simulink model "x35BusNetworkElectricityTransmissionModel"  (R2023b)
settings: Solver=VariableStepAuto  StartTime=0.0  StopTime=0.8  RelTol=1e-3
model workspace (MAT data in the model file):
  Compensation_Ki = 30
  Compensation_Kp = 3
  DC_Ki = 400
  DC_Kp = 8
  F = 0.01
  Flux_min = 0.5
  Grid_Freq_PWM = 2700
  Grid_Ireg_Ki = 5
  Grid_Ireg_Kp = 0.83
  Grid_Ireg_lim = 1.1
  Grid_Modindex_Upper = 1.1
  Grid_conv_Imax = 0.8
  H = 0.685
  Idref_max = 0.9
  Iqref_Tc = 0.3
  Ki_Var = 0.05
  Ki_Vreg = 20
  Ksh = 1.1
  L_pu = 0.3
  Llr = 0.16
  Lls = 0.18
  Lm = 2.9
  Nb_wt = 6
  P_mech = 1080000
  Pitch_Ki = 0
  Pitch_Kp = 150
  Pitch_Max = 27
  Pitch_Tc = 0.01
  Pitch_rate = 10
  Q_Filt = 50
  R_pu = 0.003
  Rotor_Freq_PWM = 1620
  Rotor_Ireg_Ki = 8
  Rotor_Ireg_Kp = 0.6
  Rotor_Ireg_lim = 0.1
  Rotor_Modindex_Upper = 2
  Rr = 0.016
  Rs = 0.023
  T_set = 0.0001
  Tp = 5e-05
  Ts = 5e-06
  Var_C_Filt = 720000
  Var_reg_max = 1.1
  Var_reg_min = 0.9
  WT_Coeff = [0.645 116 0.4 5 21 0.00912 0.08 0.035]
  WT_H = 4.32
  WT_IGBTRon = 5.931
  WT_Param = [91.204 10143]
  Wind_Freq_Filt = 10000
  Wind_Freq_nom = 60
  Wind_P_nom = 1200000
  Wind_Rotor_V_nom = 1950
  Wind_V_nom = 500
  Zeta_Filt = 0.707106781187
  init = [-0.2 0 0 0 0 0 0 0]
  p = 3
  torque0 = 0.83
  v_Ki = 0.1
  v_Kp = 3.6
  v_Max = 1.2
  v_Min = 0.7
  v_T = 5
  vreg_max = 1
  wind_VDC_nom = 1150
  wt0 = 1.2
undefined symbols (not defined in the file): D1, D11, Delta, DiscIntNeverNeededParam, Ion, Lithium, P, Q
libraries: powerlib_extras x144, spsSeriesRLCBranchLib x67, spsLoadFlowBusLib x43, spsThreePhaseTransformerTwoWindingsLib x32, spsThreePhaseSeriesRLCLoadLib x31, spsThreePhaseVIMeasurementLib x26, simulink_extras x26, spsDistributedParametersLineLib x22, spsGenericPowerSystemStabilizerLib x20, spsSynchronousMachinepuStandardLib x10, spsExcitationSystemLib x10, spsHydraulicTurbineandGovernorLib x10
(part 1 of 16)
settings Model: Creator=3.22  LastModifiedBy=3.22

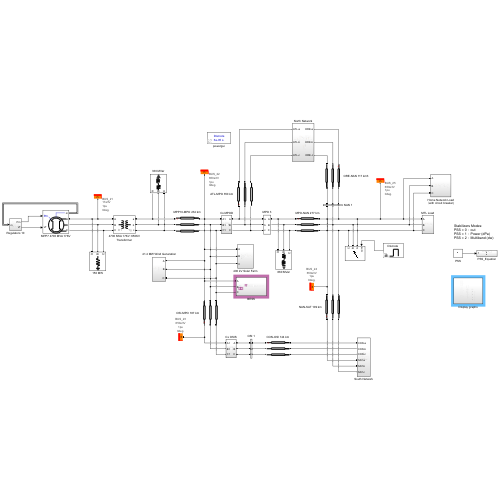
[thumbnail: Simulink's stored preview of the top-level diagram]
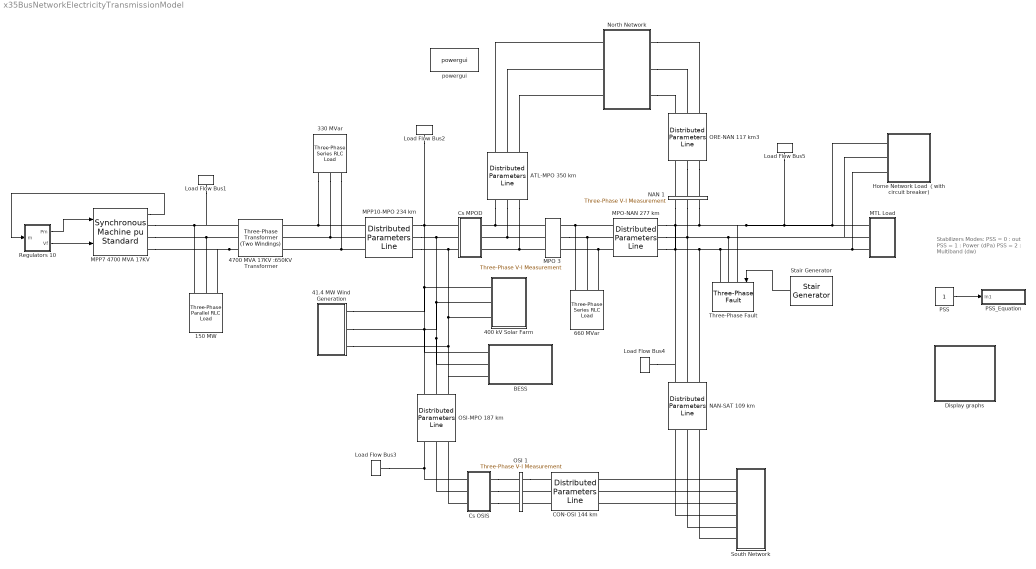
== system x35BusNetworkElectricityTransmissionModel ==
  note: Stabilizers Modes:
      | PSS = 0 :  out
      | PSS = 1 :  Power (dPa)
      | PSS = 2 :  Multiband (dw)
  " 41.4 MW Wind Generation" : Subsystem
  150 MW : spsThreePhaseParallelRLCLoadLib/Three-Phase Parallel RLC Load  LConnTagsString=A|B|C  Configuration=Y (grounded)  NominalVoltage=17000  Vabc=[1e3 1e3 1e3]  Vabcp=[1e3 1e3 1e3]  NominalFrequency=60  UnbalancedPower=off  ActivePower=150e6  InductivePower=0  CapacitivePower=0  Pabc=[10e3 9e3 11e3]  QLabc=[100 90 110]  QCabc=[100 90 110]  Pabcp=[10e3 9e3 11e3]  QLabcp=[100 90 110]  QCabcp=[100 90 110]  Measurements=None  LoadType=constant Z
  330 MVar : spsThreePhaseSeriesRLCLoadLib/Three-Phase Series RLC Load  LConnTagsString=A|B|C  Configuration=Y (grounded)  NominalVoltage=650e3  Vabc=[1e3 1e3 1e3]  Vabcp=[1e3 1e3 1e3]  NominalFrequency=60  UnbalancedPower=off  ActivePower=1100e3  InductivePower=330e6  CapacitivePower=0  Pabc=[10e3 9e3 11e3]  QLabc=[100 90 110]  QCabc=[100 90 110]  Pabcp=[10e3 9e3 11e3]  QLabcp=[100 90 110]  QCabcp=[100 90 110]  Measurements=None  LoadType=constant Z
  400 kV Solar Farm : Subsystem
  "4700 MVA 17KV :650KV Transformer " : spsThreePhaseTransformerTwoWindingsLib/Three-Phase Transformer (Two Windings)  Winding1Connection=Delta (D1)  Winding2Connection=Yg  CoreType=Three single-phase transformers  SetSaturation=off  Hysteresis=off  DataFile='hysteresis'  SetInitialFlux=off  Measurements=None  UNITS=pu  NominalPower=[ 4700e6 , 60 ]  Winding1=[ 17e3 , 0.002 , 0.08 ]  Winding2=[ 650e3 , 0.002 , 0.08 ]  Rm=500  Lm=500  L0=0.5  Saturation=[ 0,0 ; 0.0024,1.2 ; 1.0,1.52 ]  InitialFluxes=[ 0.8 , -0.8 , 0.7 ]  BreakLoop=off  DiscreteSolver=Trapezoidal iterative  DataType=off  TransfoNumber=1
  660 MVar : spsThreePhaseSeriesRLCLoadLib/Three-Phase Series RLC Load  LConnTagsString=A|B|C  Configuration=Y (grounded)  NominalVoltage=650e3  Vabc=[1e3 1e3 1e3]  Vabcp=[1e3 1e3 1e3]  NominalFrequency=60  UnbalancedPower=off  ActivePower=2200e3  InductivePower=660e6  CapacitivePower=0  Pabc=[10e3 9e3 11e3]  QLabc=[100 90 110]  QCabc=[100 90 110]  Pabcp=[10e3 9e3 11e3]  QLabcp=[100 90 110]  QCabcp=[100 90 110]  Measurements=None  LoadType=constant Z
  ATL-MPO 350 km : spsDistributedParametersLineLib/Distributed Parameters Line  Phases=3  Length=350  Frequency=60  Resistance=[0.01273 0.3864]/6  Inductance="[0.9337e-3  4.1264e-3]/6"  Capacitance=[12.74e-9 7.751e-9]*6  x1=[-0.00198 -8.81886184233511e-10 -287572.775174279 -158100.693471797;-0.00192 -9.46737266554495e-10 -283923.339530845 -164564.466267701;-0.00186 -1.01110398059622e-09 -280128.643460608 -170944.044841861;-0.0018 -1.07495339515841e-09 -276190.628400193 -177236.165283997;-0.00174 -1.13825284370079e-09 -272111.309110873 -183437.608429026;-0.00168 -1.20096994105583e-09 -267892.772647773 -189545.201504045;-0.00162 -1.26307259999766e-09 -263537.177292097 -195555.819751582;-0.00156 -1.32452904765843e-09 -259046.751446911 -201466.388028279;-0.0015 -1.38530784178394e-09 -254423.792497051 -207273.882378189;-0.00144 -1.44537788682004e-09 -249670.665633739 -212975.331579893;-0.00138 -1.50470844982173e-09 -244789.802644505 -218567.81866663;-0.00132 -1.56326917617668e-09 -239783.700669043 -224048.482418667;-0.00126 -1.62103010513521e-09 -234654.920921625 -229414.51882716;-0.0012 -1.67796168513875e-09 -229406.087380739 -234663.182528727;-0.00114 -1.73403478893901e-09 -224039.885446612 -239791.788210036;-0.00108 -1.78922072849997e-09 -218559.060567309 -244797.711981654;-0.00102 -1.84349126967524e-09 -212966.416834113 -249678.39272048;-0.00096 -1.89681864665313e-09 -207264.815546898 -254431.333380064;-0.0009 -1.94917557616222e-09 -201457.173750235 -259054.102268141;-0.00084 -2.00053527142992e-09 -195546.462740982 -263544.334290727;-0.00078 -2.05087145588711e-09 -189535.706548106 -267899.732162151;-0.00072 -2.10015837661173e-09 -183427.980385544 -272118.067580383;-0.00066 -2.1483708175044e-09 -177226.409078857 -276197.182367078;-0.0006 -2.19548411218952e-09 -170934.165466518 -280134.989571736;-0.00054 -2.24147415663495e-09 -164554.468776626 -283929.474539429;-0.00048 -2.28631742148417e-09 -158090.582979891 -287578.695941535;-0.00042 -2.32999096409427e-09 -151545.815119725 -291080.786768954;-0.00036 -2.37247244027385e-09 -144923.513620299 -294433.955287307;-0.0003 -2.41374011571475e-09 -138227.066573427 -297636.485953622;-0.00024 -2.45377287711165e-09 -131459.900005152 -300686.740294032;-0.00018 -2.49255024296411e-09 -124625.476122936 -303583.157742056;-0.00012 -2.53005237405524e-09 -117727.291544321 -306324.256437008;-6e-05 -2.56626008360181e-09 -110768.875508002 -308908.633982145]  x2=[-0.00198 1.54433518898386e-08 -267682.446603461 -181667.296939203;-0.00192 1.64654785965534e-08 -263505.082563477 -187675.172287145;-0.00186 1.74791812601711e-08 -259192.904454239 -193587.029549106;-0.0018 1.84839412516781e-08 -254748.118465748 -199399.844109673;-0.00174 1.94792445172967e-08 -250172.998632646 -205110.642025508;-0.00168 2.04645818414852e-08 -245469.885670778 -210716.501546873;-0.00162 2.14394491074616e-08 -240641.185779639 -216214.554612454;-0.00156 2.24033475551191e-08 -235689.369411317 -221601.98831671;-0.0015 2.33557840362012e-08 -230616.970006566 -226876.046349009;-0.00144 2.42962712666051e-08 -225426.582698647 -232034.030403808;-0.00138 2.52243280756855e-08 -220120.862985616 -237073.301561157;-0.00132 2.61394796524304e-08 -214702.525371715 -241991.281636816;-0.00126 2.70412577883831e-08 -209174.341978588 -246785.454501306;-0.0012 2.79292011171863e-08 -203539.141127007 -251453.367367201;-0.00114 2.88028553506256e-08 -197799.805889854 -255992.632044027;-0.00108 2.96617735110519e-08 -191959.272617088 -260400.9261601;-0.00102 3.05055161600635e-08 -186020.529433451 -264675.994350693;-0.00096 3.13336516233304e-08 -179986.614709693 -268815.649411926;-0.0009 3.21457562114475e-08 -173860.615508078 -272817.773419778;-0.00084 3.29414144367015e-08 -167645.666002995 -276680.318813656;-0.00078 3.37202192256424e-08 -161344.945877449 -280401.309443964;-0.00072 3.44817721273494e-08 -154961.67869628 -283978.84158314;-0.00066 3.52256835172862e-08 -148499.130256927 -287411.084899637;-0.0006 3.59515727966398e-08 -141960.606918587 -290696.283394352;-0.00054 3.66590685870419e-08 -135349.453910617 -293832.756299034;-0.00048 3.73478089205732e-08 -128669.053621055 -296818.898936187;-0.00042 3.80174414249525e-08 -121922.823866131 -299653.183540063;-0.00036 3.86676235038173e-08 -115114.216141641 -302334.160038285;-0.0003 3.9298022512002e-08 -108246.713857108 -304860.456793738;-0.00024 3.99083159257256e-08 -101323.830553596 -307230.781306322;-0.00018 4.04981915076007e-08 -94349.1081061232 -309443.920874218;-0.00012 4.106734746638e-08 -87326.1149115726 -311498.743214328;-6e-05 4.16154926113581e-08 -80258.4440630321 -313394.197041575]  x3=[-0.00198 -4.6655895685918e-10 -8241.46905294037 -3030.79596300684;-0.00192 -4.60608629980999e-10 -8170.81094503147 -3216.42300046448;-0.00186 -4.54422647216651e-10 -8095.97249926386 -3400.40445648242;-0.0018 -4.48004173429221e-10 -8016.99200436926 -3582.64620274818;-0.00174 -4.413564924285e-10 -7933.90986822824 -3763.05500101691;-0.00168 -4.34483005290922e-10 -7846.76859719684 -3941.53855081387;-0.00162 -4.27387228619515e-10 -7755.6127743595 -4118.00553665697;-0.00156 -4.20072792744737e-10 -7660.48903671955 -4292.36567477553;-0.0015 -4.12543439867139e-10 -7561.44605133885 -4464.52975930106;-0.00144 -4.04803022142778e-10 -7458.53449043883 -4634.40970790672;-0.00138 -3.9685549971239e-10 -7351.80700547563 -4801.91860687177;-0.00132 -3.88704938675302e-10 -7241.31820020265 -4966.97075554829;-0.00126 -3.80355509009146e-10 -7127.12460273427 -5129.4817102072;-0.0012 -3.71811482436419e-10 -7009.28463662502 -5289.36832724124;-0.00114 -3.63077230238992e-10 -6887.85859097897 -5446.54880570278;-0.00108 -3.54157221021679e-10 -6762.90858960479 -5600.94272915467;-0.00102 -3.45056018426017e-10 -6634.49855923199 -5752.4711068128;-0.00096 -3.35778278795427e-10 -6502.69419680484 -5901.05641395925;-0.0009 -3.26328748792936e-10 -6367.56293587064 -6046.62263160532;-0.00084 -3.16712262972701e-10 -6229.17391207941 -6189.09528538433;-0.00078 -3.06933741306559e-10 -6087.59792781285 -6328.401483654;-0.00072 -2.96998186666881e-10 -5942.90741596056 -6464.46995478922;-0.00066 -2.86910682267009e-10 -5795.17640286195 -6597.2310836459;-0.0006 -2.76676389060589e-10 -5644.4804704331 -6726.61694717737;-0.00054 -2.66300543101134e-10 -5490.89671749756 -6852.56134918508;-0.00048 -2.5578845286316e-10 -5334.50372034124 -6974.99985418576;-0.00042 -2.45145496526274e-10 -5175.3814925113 -7093.86982037787;-0.00036 -2.34377119223597e-10 -5013.61144387974 -7209.11043169023;-0.0003 -2.23488830255934e-10 -4849.27633899261 -7320.66272889669;-0.00024 -2.12486200273114e-10 -4682.46025472612 -7428.46963978076;-0.00018 -2.0137485842394e-10 -4513.24853727139 -7532.47600833477;-0.00012 -1.90160489476217e-10 -4341.72775846975 -7632.62862297877;-6e-05 -1.78848830908316e-10 -4167.98567152098 -7728.87624378449]  x4=[-0.00198 4.4437183156576e-10 -5640.56823399598 -1579.41875960243;-0.00192 4.46231326418624e-10 -5603.40220789252 -1706.59093166833;-0.00186 4.47862521079487e-10 -5563.36937768053 -1832.88998027941;-0.0018 4.49264580999017e-10 -5520.49022489568 -1958.25128850867;-0.00174 4.50436788857453e-10 -5474.78668730484 -2082.6107191944;-0.00168 4.51378544931595e-10 -5426.28214768235 -2205.90464775398;-0.00162 4.52089367401633e-10 -5375.00142184694 -2328.06999473533;-0.00156 4.52568892597658e-10 -5320.9707459655 -2449.04425808958;-0.0015 4.52816875185718e-10 -5264.2177631302 -2568.76554514826;-0.00144 4.52833188293339e-10 -5204.77150921571 -2687.17260428872;-0.00138 4.52617823574434e-10 -5142.662398024 -2804.20485627158;-0.00132 4.52170891213572e-10 -5077.92220572397 -2919.80242523422;-0.00126 4.51492619869608e-10 -5010.58405459429 -3033.90616932437;-0.0012 4.50583356558695e-10 -4940.68239607732 -3146.45771095815;-0.00114 4.49443566476743e-10 -4868.25299315321 -3257.39946668715;-0.00108 4.48073832761419e-10 -4793.33290204283 -3366.67467665917;-0.00102 4.46474856193802e-10 -4715.96045324916 -3474.22743365762;-0.00096 4.44647454839849e-10 -4636.17523194667 -3580.00271170466;-0.0009 4.4259256363186e-10 -4554.01805772885 -3683.94639421356;-0.00084 4.40311233890147e-10 -4469.53096372412 -3786.00530167567;-0.00078 4.37804632785159e-10 -4382.75717509091 -3886.12721886811;-0.00072 4.35074042740339e-10 -4293.74108690288 -3984.260921568;-0.00066 4.3212086077601e-10 -4202.52824143558 -4080.35620275974;-0.0006 4.28946597794631e-10 -4109.16530486617 -4174.36389832184;-0.00054 4.25552877807799e-10 -4013.70004339815 -4266.23591218018;-0.00048 4.21941437105368e-10 -3916.18129882327 -4355.92524091487;-0.00042 4.18114123367132e-10 -3816.6589635332 -4443.38599780806;-0.00036 4.14072894717521e-10 -3715.18395499364 -4528.57343632044;-0.0003 4.09819818723784e-10 -3611.808189694 -4611.44397298439;-0.00024 4.0535707133819e-10 -3506.58455658597 -4691.95520970207;-0.00018 4.00686935784761e-10 -3399.56689002456 -4770.0659554371;-0.00012 3.95811801391141e-10 -3290.80994222544 -4845.73624728864;-6e-05 3.90734162366169e-10 -3180.3693552527 -4918.92737093716]  x5=0.0019793954844851  V1=[4.219e-16 0.0001256 0.0001256;377 377 377;2.896 1.02 -0.5506]  V2=[3.447e-16 8.016e-05 8.016e-05;377 377 377;2.788 1.015 -0.5555]  I1=[4.128e-19 5.188e-07 5.188e-07;377 377 377;2.697 1.572 0.0007381]  I2=[5.884e-19 5.436e-07 5.436e-07;377 377 377;2.289 0.05248 -1.518]  nHarmo=1  Measurements=None  Decoupling=off  VsMag0=0  VrMag0=0  VsAngle0=0  VrAngle0=0  IsMag0=0  IrMag0=0  IsAngle0=0  IrAngle0=0
      settings: LibrarySourceBlock=sps_lib/Power Grid Elements/Distributed Parameters Line
  BESS : Subsystem
  CON-OSI 144 km : spsDistributedParametersLineLib/Distributed Parameters Line  Phases=3  Length=144  Frequency=60  Resistance=[0.01273 0.3864]/6  Inductance="[0.9337e-3  4.1264e-3]/6"  Capacitance=[12.74e-9 7.751e-9]*6  x1=[-0.00084 1.00465090106322e-08 0 0;-0.00078 1.0437043643029e-08 0 0;-0.00072 1.08222384910436e-08 0 0;-0.00066 1.12018964818742e-08 0 0;-0.0006 1.15758233754775e-08 0 0;-0.00054 1.19438278639452e-08 -161808.366832188 -299092.068846077;-0.00048 1.23057216693812e-08 -155002.244278101 -302675.302733702;-0.00042 1.26613196402275e-08 -148116.819711728 -306103.682343652;-0.00036 1.30104398459916e-08 -141155.615843508 -309375.45365357;-0.0003 1.33529036703253e-08 -134122.194153965 -312488.942764797;-0.00024 1.36885359024078e-08 -127020.1530716 -315442.556758774;-0.00018 1.40171648265877e-08 -119853.126131861 -318234.784512005;-0.00012 1.43386223102348e-08 -112624.780118162 -320864.197469177;-6e-05 1.46527438897608e-08 -105338.813185888 -323329.450374036]  x2=[-0.00084 1.696883336304e-08 0 0;-0.00078 1.76603541306248e-08 0 0;-0.00072 1.83428395347105e-08 0 0;-0.00066 1.90159404031536e-08 0 0;-0.0006 1.96793123651122e-08 0 0;-0.00054 2.0332616027233e-08 -156405.712657969 -298820.407534756;-0.00048 2.09755171472907e-08 -149607.117035199 -302281.515873199;-0.00042 2.16076868051928e-08 -142731.979646933 -305587.971402601;-0.00036 2.22288015712613e-08 -135783.817940495 -308738.082479218;-0.0003 2.28385436717049e-08 -128766.186723802 -311730.237448014;-0.00024 2.34366011511983e-08 -121682.676346656 -314562.905467219;-0.00018 2.40226680324841e-08 -114536.910863854 -317234.637291533;-0.00012 2.45964444729166e-08 -107332.546181055 -319744.066013586;-6e-05 2.51576369178668e-08 -100073.268184352 -322089.907763276]  x3=[-0.00084 -2.32474030583707e-10 0 0;-0.00078 -2.23427423220123e-10 0 0;-0.00072 -2.14266506258355e-10 0 0;-0.00066 -2.04995966592796e-10 0 0;-0.0006 -1.95620547202837e-10 0 0;-0.00054 -1.86145044726278e-10 -4133.07539991967 -6898.70820759528;-0.00048 -1.76574307005272e-10 -3975.98619314656 -6990.42432957894;-0.00042 -1.66913230606083e-10 -3816.86279836927 -7078.5640213074;-0.00036 -1.57166758313915e-10 -3655.78662605681 -7163.08218888573;-0.0003 -1.47339876604086e-10 -3492.84008575529 -7243.93559125769;-0.00024 -1.37437613090858e-10 -3328.10654392563 -7321.08286232862;-0.00018 -1.27465033955217e-10 -3161.67028129177 -7394.48453212913;-0.00012 -1.17427241352923e-10 -2993.61644972104 -7464.10304700863;-6e-05 -1.07329370804146e-10 -2824.03102865897 -7529.90278884852]  x4=[-0.00084 3.81260191027999e-10 0 0;-0.00078 3.81331768701559e-10 0 0;-0.00072 3.8120824999605e-10 0 0;-0.00066 3.80889698105924e-10 0 0;-0.0006 3.80376276008215e-10 0 0;-0.00054 3.79668246379155e-10 -4123.74727696322 -5625.68716163841;-0.00048 3.78765971459785e-10 -3995.45299481996 -5717.51781638891;-0.00042 3.77669912870626e-10 -3865.11456509707 -5806.42328337696;-0.00036 3.76380631375504e-10 -3732.79867134357 -5892.35807692286;-0.0003 3.74898786594656e-10 -3598.57300881562 -5975.27823119836;-0.00024 3.73225136667253e-10 -3462.50624984237 -6055.14132272033;-0.00018 3.71360537863524e-10 -3324.66800869195 -6131.90649205544;-0.00012 3.6930594414667e-10 -3185.12880595548 -6205.53446472462;-6e-05 3.67062406684801e-10 -3043.96003246747 -6275.98757129655]  x5=0.000814379856473869  V1=[3.066e-13 0.3294 0.3294;377 377 377;-0.5534 -1.851 2.861]  V2=[2.167e-13 0.2213 0.2213;377 377 377;-0.5727 -1.852 2.86]  I1=[4.19e-16 0.002316 0.002316;377 377 377;0.2564 -0.79 -2.361]  I2=[5.677e-16 0.002387 0.002387;377 377 377;-1.374 -3.038 1.674]  nHarmo=1  Measurements=None  Decoupling=off  VsMag0=0  VrMag0=0  VsAngle0=0  VrAngle0=0  IsMag0=0  IrMag0=0  IsAngle0=0  IrAngle0=0
      settings: LibrarySourceBlock=sps_lib/Power Grid Elements/Distributed Parameters Line
  Cs MPOD : Subsystem
  Cs OSIS : Subsystem
  Display graphs : Subsystem
  Home Network Load （with circuit breaker) : Subsystem
  Load Flow Bus1 : spsLoadFlowBusLib/Load Flow Bus  LConnTagsString=a  Phases=single  Connectors=on one side  ID=BUS_21  Vbase=17e3  Vref=1  Vangle=0  VLF=1  VLFb=1  VLFc=1  angleLF=0  angleLFb=0  angleLFc=0
  Load Flow Bus2 : spsLoadFlowBusLib/Load Flow Bus  LConnTagsString=a  Phases=single  Connectors=on one side  ID=BUS_22  Vbase=650e3  Vref=1  Vangle=0  VLF=1  VLFb=1  VLFc=1  angleLF=0  angleLFb=0  angleLFc=0
  Load Flow Bus3 : spsLoadFlowBusLib/Load Flow Bus  LConnTagsString=a  Phases=single  Connectors=on one side  ID=BUS_23  Vbase=650e3  Vref=1  Vangle=0  VLF=1  VLFb=1  VLFc=1  angleLF=0  angleLFb=0  angleLFc=0
  Load Flow Bus4 : spsLoadFlowBusLib/Load Flow Bus  LConnTagsString=a  Phases=single  Connectors=on one side  ID=BUS_24  Vbase=650e3  Vref=1  Vangle=0  VLF=1  VLFb=1  VLFc=1  angleLF=0  angleLFb=0  angleLFc=0
  Load Flow Bus5 : spsLoadFlowBusLib/Load Flow Bus  LConnTagsString=a  Phases=single  Connectors=on one side  ID=BUS_25  Vbase=650e3  Vref=1  Vangle=0  VLF=1  VLFb=1  VLFc=1  angleLF=0  angleLFb=0  angleLFc=0
  MPO 3 : spsThreePhaseVIMeasurementLib/Three-Phase V-I Measurement  VoltageMeasurement=no  SetLabelV=off  LabelV=Vabc_MPO3  Vpu=off  VpuLL=off  CurrentMeasurement=no  SetLabelI=off  LabelI=Iabc  Ipu=off  Pbase=100e6  Vbase=500e3  OutputType=Complex  PhasorSimulation=off  PSBequivalent=0
  MPO-NAN 277 km : spsDistributedParametersLineLib/Distributed Parameters Line  Phases=3  Length=277  Frequency=60  Resistance=[0.01273 0.3864]/6  Inductance="[0.9337e-3  4.1264e-3]/6"  Capacitance=[12.74e-9 7.751e-9]*6  x1=[-0.00162 -1.26307259999766e-09 -263537.177292097 -195555.819751582;-0.00156 -1.32452904765843e-09 -259046.751446911 -201466.388028279;-0.0015 -1.38530784178394e-09 -254423.792497051 -207273.882378189;-0.00144 -1.44537788682004e-09 -249670.665633739 -212975.331579893;-0.00138 -1.50470844982173e-09 -244789.802644505 -218567.81866663;-0.00132 -1.56326917617668e-09 -239783.700669043 -224048.482418667;-0.00126 -1.62103010513521e-09 -234654.920921625 -229414.51882716;-0.0012 -1.67796168513875e-09 -229406.087380739 -234663.182528727;-0.00114 -1.73403478893901e-09 -224039.885446612 -239791.788210036;-0.00108 -1.78922072849997e-09 -218559.060567309 -244797.711981654;-0.00102 -1.84349126967524e-09 -212966.416834113 -249678.39272048;-0.00096 -1.89681864665313e-09 -207264.815546898 -254431.333380064;-0.0009 -1.94917557616222e-09 -201457.173750235 -259054.102268141;-0.00084 -2.00053527142992e-09 -195546.462740982 -263544.334290727;-0.00078 -2.05087145588711e-09 -189535.706548106 -267899.732162151;-0.00072 -2.10015837661173e-09 -183427.980385544 -272118.067580383;-0.00066 -2.1483708175044e-09 -177226.409078857 -276197.182367078;-0.0006 -2.19548411218952e-09 -170934.165466518 -280134.989571736;-0.00054 -2.24147415663495e-09 -164554.468776626 -283929.474539429;-0.00048 -2.28631742148417e-09 -158090.582979891 -287578.695941535;-0.00042 -2.32999096409427e-09 -151545.815119725 -291080.786768954;-0.00036 -2.37247244027385e-09 -144923.513620299 -294433.955287307;-0.0003 -2.41374011571475e-09 -138227.066573427 -297636.485953622;-0.00024 -2.45377287711165e-09 -131459.900005152 -300686.740294032;-0.00018 -2.49255024296411e-09 -124625.476122936 -303583.157742056;-0.00012 -2.53005237405524e-09 -117727.291544321 -306324.256437008;-6e-05 -2.56626008360181e-09 -110768.875508002 -308908.633982145]  x2=[-0.00162 -9.4179426077037e-10 -236199.986802858 -173177.901512299;-0.00156 -1.20956811151287e-09 -232222.691432723 -178475.891100425;-0.0015 -1.47672312485927e-09 -228126.586642669 -183682.569124809;-0.00144 -1.74312261936829e-09 -223913.768075595 -188795.271752766;-0.00138 -2.00863030013604e-09 -219586.391087322 -193811.383231158;-0.00132 -2.27311032852701e-09 -215146.669643879 -198728.337224666;-0.00126 -2.53642739167166e-09 -210596.875188792 -203543.618128772;-0.0012 -2.79844677169495e-09 -205939.335480976 -208254.762356791;-0.00114 -3.05903441464048e-09 -201176.433403807 -212859.359600282;-0.00108 -3.31805699905503e-09 -196310.605745995 -217355.054062213;-0.00102 -3.57538200419821e-09 -191344.341954881 -221739.545662226;-0.00096 -3.83087777784259e-09 -186280.182862786 -226010.591213402;-0.0009 -4.08441360362934e-09 -181120.719387076 -230166.005569918;-0.00084 -4.33585976794518e-09 -175868.591204601 -234203.662745006;-0.00078 -4.58508762628627e-09 -170526.485401189 -238121.496998647;-0.00072 -4.83196966907507e-09 -165097.135096878 -241917.503894445;-0.00066 -5.07637958689664e-09 -159583.318047607 -245589.741325128;-0.0006 -5.31819233512084e-09 -153987.855224062 -249136.330506173;-0.00054 -5.5572841978775e-09 -148313.609368416 -252555.456937021;-0.00048 -5.79353285135172e-09 -142563.483529697 -255845.371329412;-0.00042 -6.02681742636701e-09 -136740.419578534 -259004.390502351;-0.00036 -6.25701857022418e-09 -130847.396702042 -262030.898243259;-0.0003 -6.48401850776443e-09 -124887.429879615 -264923.346134851;-0.00024 -6.70770110162521e-09 -118863.568340407 -267680.25434734;-0.00018 -6.92795191165833e-09 -112778.894003291 -270300.212395542;-0.00012 -7.14465825347962e-09 -106636.519900088 -272781.87986051;-6e-05 -7.35770925612033e-09 -100439.588582887 -275123.987075311]  x3=[-0.00162 1.16898131598743e-10 -5110.9747351626 -4891.8406560471;-0.00156 1.15857783477333e-10 -4999.02556707513 -5006.18778806368;-0.0015 1.14758160373091e-10 -4884.51880513618 -5117.97366190419;-0.00144 1.13599824873514e-10 -4767.51303312098 -5227.14108584998;-0.00138 1.12383369604449e-10 -4648.06811334453 -5333.63420782979;-0.00132 1.11109416926888e-10 -4526.24515603487 -5437.39854399464;-0.00126 1.09778618618562e-10 -4402.10648806799 -5538.38100659281;-0.0012 1.08391655540474e-10 -4275.71562108024 -5636.5299311305;-0.00114 1.06949237288565e-10 -4147.1372189746 -5731.79510280432;-0.00108 1.05452101830664e-10 -4016.43706483745 -5824.12778219215;-0.00102 1.03901015128935e-10 -3883.6820272827 -5913.4807301891;-0.00096 1.02296770747997e-10 -3748.9400262406 -5999.80823217593;-0.0009 1.00640189448917e-10 -3612.27999820863 -6083.06612140747;-0.00084 9.89321187692982e-11 -3473.77186098232 -6163.21180160915;-0.00078 9.71734325896615e-11 -3333.48647788401 -6240.20426877008;-0.00072 9.53650306863534e-11 -3191.49562150786 -6314.00413212138;-0.00066 9.35078382712029e-11 -3047.87193699969 -6384.57363428931;-0.0006 9.16028055181667e-11 -2902.68890489035 -6451.87667061258;-0.00054 8.96509070772022e-11 -2756.02080350175 -6515.87880761419;-0.00048 8.76531415756187e-11 -2607.94267094467 -6576.54730061822;-0.00042 8.56105311071613e-11 -2458.53026672789 -6633.85111050264;-0.00036 8.35241207090887e-11 -2307.86003299823 -6687.76091957945;-0.0003 8.1394977827513e-11 -2156.00905543135 -6738.24914659419;-0.00024 7.92241917712746e-11 -2003.05502379324 -6785.28996083701;-0.00018 7.70128731546312e-11 -1849.07619219275 -6828.85929535812;-0.00012 7.47621533290476e-11 -1694.15133904534 -6868.93485928091;-6e-05 7.24731838043751e-11 -1538.35972676856 -6905.49614920637]  x4=[-0.00162 -9.91475162198558e-11 -7334.14178280193 -1196.88834078355;-0.00156 -1.00668550134117e-10 -7305.19431472906 -1362.46270857868;-0.0015 -1.02138080157989e-10 -7272.5093742603 -1527.34001527669;-0.00144 -1.03555354452758e-10 -7236.10368361514 -1691.43590660088;-0.00138 -1.04919647914705e-10 -7195.99586861763 -1854.66642806112;-0.00132 -1.06230262546087e-10 -7152.20644916701 -2016.94806790646;-0.00126 -1.07486527812241e-10 -7104.75782873942 -2178.19779985135;-0.0012 -1.08687800984644e-10 -7053.67428292582 -2338.33312555336;-0.00114 -1.09833467469743e-10 -6998.98194701216 -2497.27211682091;-0.00108 -1.10922941123395e-10 -6940.70880260809 -2654.93345752922;-0.00102 -1.11955664550749e-10 -6878.88466333105 -2811.23648522312;-0.00096 -1.12931109391415e-10 -6813.54115955308 -2966.10123238551;-0.0009 -1.1384877658979e-10 -6744.71172221811 -3119.44846735016;-0.00084 -1.14708196650378e-10 -6672.43156573812 -3271.19973483813;-0.00078 -1.15508929877996e-10 -6596.73766997673 -3421.27739609693;-0.00072 -1.16250566602729e-10 -6517.66876132969 -3569.60466862196;-0.00066 -1.16932727389524e-10 -6435.26529291168 -3716.10566543981;-0.0006 -1.17555063232318e-10 -6349.56942385979 -3860.70543393348;-0.00054 -1.18117255732595e-10 -6260.62499776409 -4003.32999418952;-0.00048 -1.18619017262283e-10 -6168.47752023649 -4143.90637684749;-0.00042 -1.19060091110913e-10 -6073.17413562918 -4282.36266043249;-0.00036 -1.19440251616952e-10 -5974.76360291472 -4418.62800815144;-0.0003 -1.19759304283262e-10 -5873.29627074008 -4552.63270413457;-0.00024 -1.20017085876603e-10 -5768.82405166729 -4684.30818910328;-0.00018 -1.2021346451115e-10 -5661.40039561405 -4813.58709544638;-0.00012 -1.20348339715962e-10 -5551.08026250776 -4940.40328168659;-6e-05 -1.20421642486395e-10 -5437.92009416701 -5064.69186631973]  x5=0.00156655014057821  V1=[4.219e-16 0.0001256 0.0001256;377 377 377;3.052 1.115 -0.4557]  V2=[4.095e-15 0.006804 0.006804;377 377 377;-1.109 1.061 -0.5096]  I1=[9.849e-18 6.958e-05 6.958e-05;377 377 377;-2.423 -0.4689 -2.04]  I2=[7.867e-18 6.871e-05 6.871e-05;377 377 377;0.191 2.298 0.7273]  nHarmo=1  Measurements=None  Decoupling=off  VsMag0=0  VrMag0=0  VsAngle0=0  VrAngle0=0  IsMag0=0  IrMag0=0  IsAngle0=0  IrAngle0=0
      settings: LibrarySourceBlock=sps_lib/Power Grid Elements/Distributed Parameters Line
  MPP10-MPO 234 km : spsDistributedParametersLineLib/Distributed Parameters Line  Phases=3  Length=234  Frequency=60  Resistance=[0.01273 0.3864]/6  Inductance="[0.9337e-3  4.1264e-3]/6"  Capacitance=[12.74e-9 7.751e-9]*6  x1=[-0.00138 3.31492995124857e-08 -199940.184096569 -213034.098249229;-0.00132 3.3147034255945e-08 -195070.717887214 -217501.787203368;-0.00126 3.31278103641922e-08 -190101.449894095 -221858.198224203;-0.0012 3.30916376725254e-08 -185034.92248654 -226101.102491359;-0.00114 3.30385346875623e-08 -179873.727793588 -230228.329256612;-0.00108 3.29685285777711e-08 -174620.506377813 -234237.766954486;-0.00102 3.28816551595711e-08 -169277.945884359 -238127.364282571;-0.00096 3.27779588790084e-08 -163848.779665894 -241895.131251001;-0.0009 3.26574927890161e-08 -158335.785384174 -245539.140200574;-0.00084 3.25203185222719e-08 -152741.783588943 -249057.52678898;-0.00078 3.23665062596653e-08 -147069.636274884 -252448.490944626;-0.00072 3.2196134694392e-08 -141322.245417373 -255710.297787593;-0.00066 3.20092909916928e-08 -135502.551487771 -258841.278517229;-0.0006 3.18060707442586e-08 -129613.531949028 -261839.831265939;-0.00054 3.15865779233231e-08 -123658.199732358 -264704.421918729;-0.00048 3.13509248254691e-08 -117639.601695764 -267433.58489809;-0.00042 3.10992320151759e-08 -111560.817065213 -270025.923913813;-0.00036 3.0831628263136e-08 -105424.955859244 -272480.112677356;-0.0003 3.05482504803737e-08 -99235.1572978279 -274794.8955804;-0.00024 3.02492436481989e-08 -92994.5881962837 -276969.088337239;-0.00018 2.99347607440319e-08 -86706.4413450759 -279001.578590685;-0.00012 2.96049626631375e-08 -80373.933876325 -280891.326481167;-6e-05 2.92600181363078e-08 -74000.3056178636 -282637.365178746]  x2=[-0.00138 1.63037176569151e-09 -239783.980582736 -223567.755994609;-0.00132 1.60101071654693e-09 -234666.073998373 -228933.921650626;-0.00126 1.57083056073649e-09 -229428.107914421 -234182.960482113;-0.0012 1.53984673898556e-09 -224072.762171116 -239312.186983814;-0.00114 1.50807510318988e-09 -218602.776662296 -244318.976948674;-0.00108 1.47553190830537e-09 -213020.949933621 -249200.768810431;-0.00102 1.44223380403188e-09 -207330.137750785 -253955.064954163;-0.00096 1.40819782629484e-09 -201533.251638455 -258579.432994115;-0.0009 1.37344138852935e-09 -195633.257390681 -263071.507018149;-0.00084 1.33798227277122e-09 -189633.173553539 -267428.98879819;-0.00078 1.30183862055927e-09 -183536.069880788 -271649.648966042;-0.00072 1.26502892365382e-09 -177345.06576333 -275731.328153974;-0.00066 1.22757201457599e-09 -171063.328633268 -279671.938099494;-0.0006 1.18948705697258e-09 -164694.072343389 -283469.462713739;-0.00054 1.15079353581163e-09 -158240.555522904 -287121.959112946;-0.00048 1.11151124741353e-09 -151706.079910263 -290627.558612467;-0.00042 1.07166028932289e-09 -145093.988663934 -293984.467682822;-0.00036 1.03126105002624e-09 -138407.664651977 -297190.968867303;-0.0003 9.90334198520868e-10 -131650.528721303 -300245.421660653;-0.00024 9.48900673740267e-10 -124826.037947514 -303146.263348384;-0.00018 9.06981673841311e-10 -117937.683866191 -305892.009806287;-0.00012 8.64598645358924e-10 -110988.990686564 -308481.256259738;-6e-05 8.21773272233625e-10 -103983.513488461 -310912.678002409]  x3=[-0.00138 1.59320603146652e-10 -5992.3721084524 -1106.47016711861;-0.00132 1.49790850655811e-10 -5965.81298347456 -1241.72026897558;-0.00126 1.40184462397958e-10 -5936.20163833882 -1376.33508379858;-0.0012 1.30506353178831e-10 -5903.55322275652 -1510.24574016097;-0.00114 1.20761474497938e-10 -5867.88444026033 -1643.38372689655;-0.00108 1.10954812015276e-10 -5829.21353965847 -1775.68092815122;-0.00102 1.01091383000578e-10 -5787.56030569824 -1907.06965823223;-0.00096 9.11762337663825e-11 -5742.94604894379 -2037.4826962375;-0.0009 8.12144370862493e-11 -5695.39359487326 -2166.85332044701;-0.00084 7.12110895994325e-11 -5644.92727220082 -2295.11534245895;-0.00078 6.1171309203347e-11 -5591.57290042966 -2422.20314105282;-0.00072 5.11002324351573e-11 -5535.35777664225 -2548.05169576257;-0.00066 4.100301184383e-11 -5476.31066153466 -2672.59662014218;-0.0006 3.08848133539948e-11 -5414.46176470204 -2795.77419470701;-0.00054 2.0750813622962e-11 -5349.84272918285 -2917.52139953387;-0.00048 1.06061973922488e-11 -5282.48661526969 -3037.77594650313;-0.00042 4.56154834969669e-13 -5212.42788359502 -3156.47631116651;-0.00036 -9.6941210995518e-12 -5139.70237750051 -3273.56176422413;-0.0003 -1.9839437342592e-11 -5064.34730469889 -3388.9724025947;-0.00024 -2.9974603362897e-11 -4986.40121823781 -3502.64918006309;-0.00018 -4.00944338222546e-11 -4905.90399677538 -3614.53393748945;-0.00012 -5.01937512284088e-11 -4822.89682417751 -3724.56943256448;-6e-05 -6.02673885839606e-11 -4737.42216844751 -3832.69936909568]  x4=[-0.00138 1.06140237550058e-10 -5148.01117264408 -7003.97229448765;-0.00132 1.1689708808364e-10 -4988.28140964082 -7118.61680752999;-0.00126 1.27594131906949e-10 -4825.99954969555 -7229.61930467669;-0.0012 1.38225896214705e-10 -4661.24861920643 -7336.92299499911;-0.00114 1.48786941599837e-10 -4494.11290779376 -7440.47297994653;-0.00108 1.5927186483638e-10 -4324.6779251758 -7540.21628143329;-0.00102 1.69675301643868e-10 -4153.03035742046 -7636.10186894328;-0.00096 1.79991929431794e-10 -3979.25802259509 -7728.08068563818;-0.0009 1.90216470022756e-10 -3803.44982583712 -7816.1056734558;-0.00084 2.00343692352857e-10 -3625.69571386858 -7900.13179718585;-0.00078 2.10368415148025e-10 -3446.08662897767 -7980.11606751081;-0.00072 2.20285509574841e-10 -3264.71446249102 -8056.01756300004;-0.00066 2.30089901864551e-10 -3081.67200776037 -8127.79745104595;-0.0006 2.39776575908895e-10 -2897.0529126878 -8195.41900773148;-0.00054 2.49340575826442e-10 -2710.95163181372 -8258.84763661872;-0.00048 2.58777008498112e-10 -2523.46337799217 -8318.05088644911;-0.00042 2.68081046070585e-10 -2334.6840736782 -8372.99846774607;-0.00036 2.7724792842632e-10 -2144.71030185213 -8423.66226831173;-0.0003 2.86272965618919e-10 -1953.63925660595 -8470.01636760952;-0.00024 2.95151540272592e-10 -1761.56869341698 -8512.03705002574;-0.00018 3.03879109944488e-10 -1568.59687913442 -8549.70281700281;-0.00012 3.12451209448696e-10 -1374.82254170415 -8582.99439803836;-6e-05 3.20863453140715e-10 -1180.34481965774 -8611.89476054436]  x5=0.00132336726677004  V1=[5.094e-16 1.649e-05 1.649e-05;377 377 377;1.389 -1.935 2.777]  V2=[3.793e-13 0.4417 0.4417;377 377 377;-0.7025 -1.967 2.745]  I1=[9.917e-16 0.005412 0.005412;377 377 377;-2.043 2.781 1.21]  I2=[8.773e-16 0.005353 0.005353;377 377 377;0.5828 -0.6661 -2.237]  nHarmo=1  Measurements=None  Decoupling=off  VsMag0=0  VrMag0=0  VsAngle0=0  VrAngle0=0  IsMag0=0  IrMag0=0  IsAngle0=0  IrAngle0=0
      settings: LibrarySourceBlock=sps_lib/Power Grid Elements/Distributed Parameters Line
  MPP7 4700 MVA 17KV : spsSynchronousMachinepuStandardLib/Synchronous Machine pu Standard  PresetModel=No  MechanicalLoad=Mechanical power Pm  ShowDetailedParameters=on  RotorType=Salient-pole  Units=per unit standard parameters  MeasurementBus=off  NominalParameters=[2700e6 17000 60]  Reactances1=[ 1.81, 0.3, 0.23, 1.76, 0.65, 0.25, 0.15 ]  Reactances2=[ 1.305, 0.296, 0.252, 0.474, 0.243, 0.18 ]  dAxisTimeConstants=Short-circuit  qAxisTimeConstants=Open-circuit  TimeConstants1="[ 4.4849  0.0681  0.1  ]"  TimeConstants2=[ 8.0, 0.03, 1.0, 0.07 ]  TimeConstants3="[  4.49  0.0681  0.0513  ]"  TimeConstants4=[ 8.0, 0.03, 0.3371, 0.0295 ]  TimeConstants5=[ 1.01, 0.053, 0.1 ]  TimeConstants6=[ 1.3201, 0.023, 1.0, 0.07 ]  TimeConstants7=[0.012 0.003 0.003]  TimeConstants8=[ 1.3201, 0.0231, 0.3371, 0.0295 ]  StatorResistance=2.8544e-3  Mechanical=[3.5 0 32]  PolePairs=20  InitialConditions=[0 -81.9543 0.907703 0.907703 0.907703 -8.76021 -128.76 111.24 1.25655]  SetSaturation=off  Saturation=[0.6404,0.7127,0.8441,0.9214,0.9956,1.082,1.19,1.316,1.457;0.7,0.7698,0.8872,0.9466,0.9969,1.046,1.1,1.151,1.201]  LoadFlowParameters=[1,0,0,0,0]  TsPowergui=0  TsBlock=-1  IterativeModel=Trapezoidal non iterative  IterativeDiscreteModel=Trapezoidal non iterative  BusType=PV  Pref=3845e6  Qref=0  Qmin=-inf  Qmax=inf  PLF=0  QLF=0
  MTL Load : Subsystem
  NAN 1 : spsThreePhaseVIMeasurementLib/Three-Phase V-I Measurement  VoltageMeasurement=phase-to-ground  SetLabelV=on  LabelV=Vabc_NAN1  Vpu=off  VpuLL=off  CurrentMeasurement=no  SetLabelI=off  LabelI=Iabc  Ipu=off  Pbase=100e6  Vbase=500e3  OutputType=Complex  PhasorSimulation=off  PSBequivalent=0
  NAN-SAT 109 km : spsDistributedParametersLineLib/Distributed Parameters Line  Phases=3  Length=109  Frequency=60  Resistance=[0.01273 0.3864]/6  Inductance="[0.9337e-3  4.1264e-3]/6"  Capacitance=[12.74e-9 7.751e-9]*6  x1=[-0.00066 2.79067720326726e-08 0 0;-0.0006 2.90655176855074e-08 0 0;-0.00054 3.02093928824253e-08 0 0;-0.00048 3.13378123957392e-08 0 0;-0.00042 3.24501989051752e-08 -79011.1892595523 -247649.579204249;-0.00036 3.35459832932406e-08 -73389.754995002 -249373.295946779;-0.0003 3.46246049363947e-08 -67730.7731757095 -250969.428703214;-0.00024 3.56855119918741e-08 -62037.1390413396 -252437.160862542;-0.00018 3.67281616800261e-08 -56311.7655603216 -253775.74150587;-0.00012 3.77520205620042e-08 -50557.5819395211 -254984.485790608;-6e-05 3.87565648126856e-08 -44777.5321256037 -256062.775300843]  x2=[-0.00066 -5.07637958689664e-09 0 0;-0.0006 -5.31819233512084e-09 0 0;-0.00054 -5.5572841978775e-09 0 0;-0.00048 -5.79353285135172e-09 0 0;-0.00042 -6.02681742636701e-09 -136740.419578534 -259004.390502351;-0.00036 -6.25701857022418e-09 -130847.396702042 -262030.898243259;-0.0003 -6.48401850776443e-09 -124887.429879615 -264923.346134851;-0.00024 -6.70770110162521e-09 -118863.568340407 -267680.25434734;-0.00018 -6.92795191165833e-09 -112778.894003291 -270300.212395542;-0.00012 -7.14465825347962e-09 -106636.519900088 -272781.87986051;-6e-05 -7.35770925612033e-09 -100439.588582887 -275123.987075311]  x3=[-0.00066 1.94219343152259e-09 0 0;-0.0006 1.91576183230784e-09 0 0;-0.00054 1.88835009394048e-09 0 0;-0.00048 1.85997224077235e-09 0 0;-0.00042 1.83064279143751e-09 -4232.75966789101 3615.63307862765;-0.00036 1.80037675142419e-09 -4313.4531717761 3518.97337966064;-0.0003 1.76918960539769e-09 -4391.93983331506 3420.51330888943;-0.00024 1.73709730927822e-09 -4468.17949728158 3320.30324030558;-0.00018 1.70411628207744e-09 -4542.13315805482 3218.39444323184;-0.00012 1.67026339749831e-09 -4613.76297957544 3114.83905609185;-6e-05 1.6355559753021e-09 -4683.03231470316 3009.69005973516]  x4=[-0.00066 -1.80450370308848e-09 0 0;-0.0006 -1.7703386889303e-09 0 0;-0.00054 -1.73526793678677e-09 0 0;-0.00048 -1.69930938950271e-09 0 0;-0.00042 -1.66248144413536e-09 -1325.62478319595 -14463.0056681374;-0.00036 -1.62480294254206e-09 -998.168425453836 -14489.2894299526;-0.0003 -1.58629316174045e-09 -670.201386301232 -14508.1602035643;-0.00024 -1.54697180404596e-09 -341.891459735499 -14519.6083343358;-0.00018 -1.50685898699178e-09 -13.4066151815367 -14523.6279651919;-0.00012 -1.46597523303629e-09 315.085088444478 -14520.2170396153;-6e-05 -1.42434145906348e-09 643.415588717141 -14509.3773026985]  x5=0.000616440308025359  V1=[4.327e-18 2.694e-07 2.694e-07;377 377 377;-0.06841 1.312 -0.2585]  V2=[4.095e-15 0.006804 0.006804;377 377 377;-0.7508 1.28 -0.2912]  I1=[2.296e-17 0.0001774 0.0001774;377 377 377;-2.081 -0.2552 -1.826]  I2=[2.168e-17 0.0001764 0.0001764;377 377 377;0.8233 2.744 1.174]  nHarmo=1  Measurements=None  Decoupling=off  VsMag0=0  VrMag0=0  VsAngle0=0  VrAngle0=0  IsMag0=0  IrMag0=0  IsAngle0=0  IrAngle0=0
      settings: LibrarySourceBlock=sps_lib/Power Grid Elements/Distributed Parameters Line
  North Network : Subsystem
  ORE-NAN 117 km3 : spsDistributedParametersLineLib/Distributed Parameters Line  Phases=3  Length=117  Frequency=60  Resistance=[0.01273 0.3864]/6  Inductance="[0.9337e-3  4.1264e-3]/6"  Capacitance=[12.74e-9 7.751e-9]*6  x1=[-0.00072 2.07278827110993e-08 0 0;-0.00066 2.0970233564842e-08 0 0;-0.0006 2.12018556596076e-08 0 0;-0.00054 2.14226304932525e-08 0 0;-0.00048 2.16324451132923e-08 0 0;-0.00042 2.18311921746906e-08 -95889.8655381057 -247719.952162324;-0.00036 2.20187699947782e-08 -90262.5207740761 -249825.405434422;-0.0003 2.21950826052764e-08 -84588.9960365589 -251803.043412857;-0.00024 2.23600398013958e-08 -78872.1940056444 -253651.854301496;-0.00018 2.25135571879867e-08 -73115.0395028861 -255370.892214528;-0.00012 2.26555562227176e-08 -67320.4779949075 -256959.277660391;-6e-05 2.27859642562584e-08 -61491.4740864473 -258416.197991741]  x2=[-0.00072 -4.83196966907507e-09 0 0;-0.00066 -5.07637958689664e-09 0 0;-0.0006 -5.31819233512084e-09 0 0;-0.00054 -5.5572841978775e-09 0 0;-0.00048 -5.79353285135172e-09 0 0;-0.00042 -6.02681742636701e-09 -136740.419578534 -259004.390502351;-0.00036 -6.25701857022418e-09 -130847.396702042 -262030.898243259;-0.0003 -6.48401850776443e-09 -124887.429879615 -264923.346134851;-0.00024 -6.70770110162521e-09 -118863.568340407 -267680.25434734;-0.00018 -6.92795191165833e-09 -112778.894003291 -270300.212395542;-0.00012 -7.14465825347962e-09 -106636.519900088 -272781.87986051;-6e-05 -7.35770925612033e-09 -100439.588582887 -275123.987075311]  x3=[-0.00072 6.26747200630813e-10 0 0;-0.00066 6.07719568620991e-10 0 0;-0.0006 5.88381016050495e-10 0 0;-0.00054 5.68741436880157e-10 0 0;-0.00048 5.48810879081578e-10 0 0;-0.00042 5.28599539496401e-10 -4391.59747935055 585.101817719601;-0.00036 5.08117758619422e-10 -4403.70726176259 485.624637123376;-0.0003 4.87376015308196e-10 -4413.56402616836 385.899001989487;-0.00024 4.66384921421865e-10 -4421.16272966506 285.975933795586;-0.00018 4.45155216391933e-10 -4426.49948461556 185.906555029729;-0.00012 4.23697761727771e-10 -4429.57156063743 85.7420630351592;-6e-05 4.02023535459675e-10 -4430.3773859998 -14.46629618319]  x4=[-0.00072 -4.97159698036882e-10 0 0;-0.00066 -4.7775319307751e-10 0 0;-0.0006 -4.58102260756695e-10 0 0;-0.00054 -4.38216954854521e-10 0 0;-0.00048 -4.18107449060925e-10 0 0;-0.00042 -3.97784031770652e-10 -1596.50446523857 -11377.5533327472;-0.00036 -3.77257100819521e-10 -1338.76405041833 -11410.7528211921;-0.0003 -3.56537158164701e-10 -1080.33869917238 -11438.1143576472;-0.00024 -3.35634804511715e-10 -821.360626685569 -11459.6239434449;-0.00018 -3.14560733890923e-10 -561.962330925148 -11475.2705738836;-0.00012 -2.93325728186258e-10 -302.276524852355 -11485.0462438581;-6e-05 -2.71940651619017e-10 -42.43606852402 -11488.9459519549]  x5=0.000661683633385019  V1=[2.771e-15 0.004375 0.004375;377 377 377;-0.7831 1.268 -0.3032]  V2=[4.095e-15 0.006804 0.006804;377 377 377;-0.7678 1.269 -0.3016]  I1=[9.029e-18 6.296e-05 6.296e-05;377 377 377;-1.689 -0.005215 -1.576]  I2=[6.955e-18 6.141e-05 6.141e-05;377 377 377;0.2743 2.461 0.89]  nHarmo=1  Measurements=None  Decoupling=off  VsMag0=0  VrMag0=0  VsAngle0=0  VrAngle0=0  IsMag0=0  IrMag0=0  IsAngle0=0  IrAngle0=0
      settings: LibrarySourceBlock=sps_lib/Power Grid Elements/Distributed Parameters Line
  OSI 1 : spsThreePhaseVIMeasurementLib/Three-Phase V-I Measurement  VoltageMeasurement=no  SetLabelV=on  LabelV=Vabc  Vpu=off  VpuLL=off  CurrentMeasurement=no  SetLabelI=off  LabelI=Iabc  Ipu=off  Pbase=100e6  Vbase=500e3  OutputType=Complex  PhasorSimulation=off  PSBequivalent=0
  OSI-MPO 187 km : spsDistributedParametersLineLib/Distributed Parameters Line  Phases=3  Length=187  Frequency=60  Resistance=[0.01273 0.3864]/6  Inductance="[0.9337e-3  4.1264e-3]/6"  Capacitance=[12.74e-9 7.751e-9]*6  x1=[-0.00108 9.68973336779815e-09 0 0;-0.00102 1.01344600887177e-08 0 0;-0.00096 1.05740018325927e-08 0 0;-0.0009 1.10081337217449e-08 0 0;-0.00084 1.14366336462783e-08 0 0;-0.00078 1.18592823777134e-08 0 0;-0.00072 1.22758636811498e-08 0 0;-0.00066 1.26861644258951e-08 -173683.36881338 -294562.604019707;-0.0006 1.30899746945067e-08 -166976.652478384 -298415.579895744;-0.00054 1.34870878901896e-08 -160184.507802607 -302115.880847021;-0.00048 1.38773008424952e-08 -153310.409772768 -305661.613731197;-0.00042 1.42604139112668e-08 -146357.875304439 -309050.964485811;-0.00036 1.46362310887792e-08 -139330.461442721 -312282.199056389;-0.0003 1.50045601000201e-08 -132231.763542399 -315353.664283618;-0.00024 1.53652125010614e-08 -125065.413428486 -318263.788749133;-0.00018 1.57180037754708e-08 -117835.07753812 -321011.083579486;-0.00012 1.60627534287132e-08 -110544.455044743 -323594.143207877;-6e-05 1.6399285080496e-08 -103197.275965539 -326011.64609327]  x2=[-0.00108 1.47553190830537e-09 0 0;-0.00102 1.44223380403188e-09 0 0;-0.00096 1.40819782629484e-09 0 0;-0.0009 1.37344138852935e-09 0 0;-0.00084 1.33798227277122e-09 0 0;-0.00078 1.30183862055927e-09 0 0;-0.00072 1.26502892365382e-09 0 0;-0.00066 1.22757201457599e-09 -171063.328633268 -279671.938099494;-0.0006 1.18948705697258e-09 -164694.072343389 -283469.462713739;-0.00054 1.15079353581163e-09 -158240.555522904 -287121.959112946;-0.00048 1.11151124741353e-09 -151706.079910263 -290627.558612467;-0.00042 1.07166028932289e-09 -145093.988663934 -293984.467682822;-0.00036 1.03126105002624e-09 -138407.664651977 -297190.968867303;-0.0003 9.90334198520868e-10 -131650.528721303 -300245.421660653;-0.00024 9.48900673740267e-10 -124826.037947514 -303146.263348384;-0.00018 9.06981673841311e-10 -117937.683866191 -305892.009806287;-0.00012 8.64598645358924e-10 -110988.990686564 -308481.256259738;-6e-05 8.21773272233625e-10 -103983.513488461 -310912.678002409]  x3=[-0.00108 4.10794168021694e-10 0 0;-0.00102 4.08721115226045e-10 0 0;-0.00096 4.06438953155549e-10 0 0;-0.0009 4.03948849406491e-10 0 0;-0.00084 4.01252077961959e-10 0 0;-0.00078 3.98350018540056e-10 0 0;-0.00072 3.95244155888006e-10 0 0;-0.00066 3.91936079022532e-10 -3246.47657687035 -6208.2508203112;-0.0006 3.88427480416883e-10 -3105.23066701941 -6280.09076957344;-0.00054 3.84720155134939e-10 -2962.39606378115 -6348.71770835523;-0.00048 3.80815999912817e-10 -2818.04584397788 -6414.09652584662;-0.00042 3.76717012188468e-10 -2672.25385984933 -6476.1937730365;-0.00036 3.72425289079754e-10 -2525.0947012685 -6534.9776798258;-0.0003 3.67943026311518e-10 -2376.64365758012 -6590.41817128159;-0.00024 3.63272517092216e-10 -2226.9766790812 -6642.48688302403;-0.00018 3.58416150940666e-10 -2076.17033816346 -6691.15717573807;-0.00012 3.53376412463525e-10 -1924.3017901375 -6736.40414880263;-6e-05 3.48155880084122e-10 -1771.4487337587 -6778.20465303023]  x4=[-0.00108 -3.53267058025546e-10 0 0;-0.00102 -3.47700212470081e-10 0 0;-0.00096 -3.41955477061155e-10 0 0;-0.0009 -3.36035790911554e-10 0 0;-0.00084 -3.29944182642095e-10 0 0;-0.00078 -3.23683768832129e-10 0 0;-0.00072 -3.1725775242504e-10 0 0;-0.00066 -3.1066942108956e-10 -5891.82469555518 -5505.17124350509;-0.0006 -3.03922145537741e-10 -5765.80372076254 -5637.0223558898;-0.00054 -2.97019377800429e-10 -5636.83285424655 -5765.98946347703;-0.00048 -2.89964649461147e-10 -5504.97807988563 -5892.00658431152;-0.00042 -2.82761569849271e-10 -5370.30685701874 -6015.00924570571;-0.00036 -2.75413824193426e-10 -5232.88808593194 -6134.93451722521;-0.0003 -2.67925171736062e-10 -5092.79207260772 -6251.72104288513;-0.00024 -2.60299443810149e-10 -4950.09049275518 -6365.309072541;-0.00018 -2.52540541879003e-10 -4804.85635513939 -6475.64049245796;-0.00012 -2.44652435540218e-10 -4657.16396422877 -6582.65885504291;-6e-05 -2.36639160494754e-10 -4507.08888217956 -6686.30940772406]  x5=0.00105756273028204  V1=[3.05e-13 0.3186 0.3186;377 377 377;-0.6471 -1.909 2.804]  V2=[3.793e-13 0.4417 0.4417;377 377 377;-0.6023 -1.906 2.806]  I1=[5.824e-16 0.002377 0.002377;377 377 377;-1.191 -2.924 1.788]  I2=[4.03e-16 0.002279 0.002279;377 377 377;-0.283 -1.078 -2.649]  nHarmo=1  Measurements=None  Decoupling=off  VsMag0=0  VrMag0=0  VsAngle0=0  VrAngle0=0  IsMag0=0  IrMag0=0  IsAngle0=0  IrAngle0=0
      settings: LibrarySourceBlock=sps_lib/Power Grid Elements/Distributed Parameters Line
  PSS : Constant
  PSS_Equation : Subsystem
  Regulators 10 : Subsystem
  South Network : Subsystem
  Stair Generator : eeStairGenerator/Stair Generator  LabelModeActiveChoice=Discrete  TimeInput=[0.1 0.15 0.2]  AmplitudeInput=[0 1 0]  SampleTime=-1  RepeatPattern=off  OutDataTypeStr=double
      settings: LibrarySourceBlock=ee_sl_lib/General Control/Stair Generator
  Three-Phase Fault : spsThreePhaseFaultLib/Three-Phase Fault  InitialStates=0  FaultA=on  FaultB=on  FaultC=on  GroundFault=on  SwitchTimes="[0.2  0.4]"  External=on  SwitchStatus=NaN  FaultResistance=0.001  GroundResistance=0.01  SnubberResistance=1e6  SnubberCapacitance=inf  Measurements=None
  powergui : sps_lib/powergui  Priority=1  SimulationMode=Discrete  SampleTime=6e-5  frequency=60  Iterations=50  frequencyindice=0  Pbase=100e6  ErrMax=1e-4  UnitsV=kV  UnitsW=MW  buscounter=0  FunctionMessages=off  echomessages=off  EnableUseOfTLC=off  CurrentSourceSwitches=off  DisableSnubberDevices=off  DisableRonSwitches=off  DisableVfSwitches=off  DisplayEquations=off  AutomaticDiscreteSolvers=off  SolverType=Tustin/Backward Euler (TBE)  Interpol=off  ExternalGateDelay=off  methode=off  Ts=100  x0status=blocks  SPID=on  SwTol=0  HookPort=off  NonlinearTolerance=1e-4  nMaxIteration=100  ContinueOnMaxIteration=off  RestoreLinks=warning  ResistiveCurrentMeasurement=off  Frange=[0:2:500]  Ylog=off  Xlog=on  ShowGrid=off  save=off  variable=ZData  structure=0  ZoomFFT=off  StartTime=0.0  cycles=1  DisplayStyle=1  fundamental=60  FreqAxis=off  MaxFrequency=1000  frequencyindicesteady=1  RmsSteady=1  display=off
  wires:
  PSS/1 -> PSS_Equation/1(In1)
  Regulators 10/1(Pm) -> MPP7 4700 MVA 17KV/1
  MPP7 4700 MVA 17KV/1 -> Regulators 10/1(m)
  Regulators 10/2(Vf) -> MPP7 4700 MVA 17KV/2
  Stair Generator/1 -> Three-Phase Fault/1
  connections:
  South Network/LConn3 -- CON-OSI 144 km/RConn3
  South Network/LConn2 -- CON-OSI 144 km/RConn2
  South Network/LConn1 -- CON-OSI 144 km/RConn1
  OSI 1/LConn1 -- CON-OSI 144 km/LConn1
  CON-OSI 144 km/LConn2 -- OSI 1/LConn2
  CON-OSI 144 km/LConn3 -- OSI 1/LConn3
  Cs OSIS/LConn1 -- OSI 1/RConn1
  Cs OSIS/LConn2 -- OSI 1/RConn2
  Cs OSIS/LConn3 -- OSI 1/RConn3
  150 MW/LConn1 -- MPP7 4700 MVA 17KV/RConn1 -- "4700 MVA 17KV :650KV Transformer "/LConn1 -- Load Flow Bus1/LConn1
  150 MW/LConn2 -- MPP7 4700 MVA 17KV/RConn2 -- "4700 MVA 17KV :650KV Transformer "/LConn2
  "4700 MVA 17KV :650KV Transformer "/LConn3 -- MPP7 4700 MVA 17KV/RConn3 -- 150 MW/LConn3
  North Network/RConn1 -- ATL-MPO 350 km/RConn1
  Cs OSIS/RConn1 -- Load Flow Bus3/LConn1 -- OSI-MPO 187 km/LConn1
  Cs OSIS/RConn2 -- OSI-MPO 187 km/LConn2
  Cs OSIS/RConn3 -- OSI-MPO 187 km/LConn3
  MPP10-MPO 234 km/LConn1 -- 330 MVar/LConn1 -- "4700 MVA 17KV :650KV Transformer "/RConn1
  MPP10-MPO 234 km/LConn2 -- 330 MVar/LConn2 -- "4700 MVA 17KV :650KV Transformer "/RConn2
  MPP10-MPO 234 km/LConn3 -- "4700 MVA 17KV :650KV Transformer "/RConn3 -- 330 MVar/LConn3
  MPP10-MPO 234 km/RConn1 -- BESS/LConn1 -- OSI-MPO 187 km/RConn1 -- " 41.4 MW Wind Generation"/LConn1 -- 400 kV Solar Farm/LConn1 -- Cs MPOD/RConn1 -- Load Flow Bus2/LConn1
  MPP10-MPO 234 km/RConn2 -- BESS/LConn2 -- OSI-MPO 187 km/RConn2 -- " 41.4 MW Wind Generation"/LConn2 -- 400 kV Solar Farm/LConn2 -- Cs MPOD/RConn2
  MPP10-MPO 234 km/RConn3 -- BESS/LConn3 -- OSI-MPO 187 km/RConn3 -- " 41.4 MW Wind Generation"/LConn3 -- 400 kV Solar Farm/LConn3 -- Cs MPOD/RConn3
  MPO 3/RConn1 -- ATL-MPO 350 km/LConn1 -- Cs MPOD/LConn1
  MPO 3/RConn2 -- ATL-MPO 350 km/LConn2 -- Cs MPOD/LConn2
  MPO 3/RConn3 -- ATL-MPO 350 km/LConn3 -- Cs MPOD/LConn3
  NAN 1/LConn2 -- Home Network Load （with circuit breaker)/LConn2 -- MTL Load/LConn2 -- Three-Phase Fault/LConn2 -- NAN-SAT 109 km/RConn2 -- MPO-NAN 277 km/RConn2
  MTL Load/LConn1 -- Home Network Load （with circuit breaker)/LConn1 -- Load Flow Bus5/LConn1 -- Three-Phase Fault/LConn1 -- Load Flow Bus4/LConn1 -- NAN-SAT 109 km/RConn1 -- MPO-NAN 277 km/RConn1 -- NAN 1/LConn1
  ATL-MPO 350 km/RConn2 -- North Network/RConn2
  North Network/RConn3 -- ATL-MPO 350 km/RConn3
  North Network/LConn1 -- ORE-NAN 117 km3/LConn1
  North Network/LConn2 -- ORE-NAN 117 km3/LConn2
  North Network/LConn3 -- ORE-NAN 117 km3/LConn3
  NAN 1/RConn3 -- ORE-NAN 117 km3/RConn3
  ORE-NAN 117 km3/RConn2 -- NAN 1/RConn2
  ORE-NAN 117 km3/RConn1 -- NAN 1/RConn1
  South Network/LConn4 -- NAN-SAT 109 km/LConn1
  South Network/LConn5 -- NAN-SAT 109 km/LConn2
  South Network/LConn6 -- NAN-SAT 109 km/LConn3
  MPO-NAN 277 km/LConn3 -- 660 MVar/LConn3 -- MPO 3/LConn3
  MPO 3/LConn2 -- 660 MVar/LConn2 -- MPO-NAN 277 km/LConn2
  MPO-NAN 277 km/LConn1 -- 660 MVar/LConn1 -- MPO 3/LConn1
  MPO-NAN 277 km/RConn3 -- NAN-SAT 109 km/RConn3 -- Home Network Load （with circuit breaker)/LConn3 -- MTL Load/LConn3 -- Three-Phase Fault/LConn3 -- NAN 1/LConn3
